simulink model "ControllerSimu"  (R2025b)
settings: Solver=VariableStepAuto  StartTime=0.0  StopTime=10.0  RelTol=1e-3
undefined symbols (not defined in the file or in its folder): a, b, delta_bp, Iz, TWFront, TWRear, U_bp, WheelRadius, Yaw_table
settings Model: Creator=ATuck  LastModifiedBy=ATuck

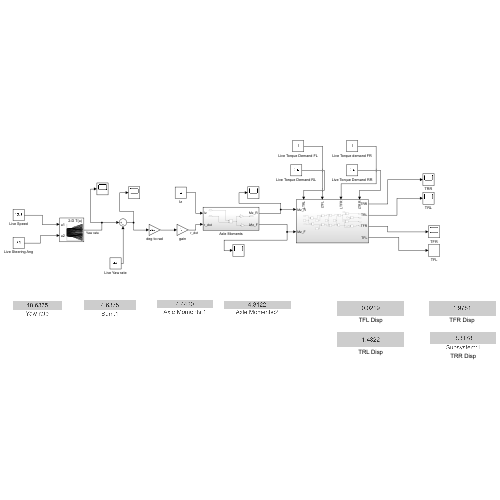
[thumbnail: Simulink's stored preview of the top-level diagram]
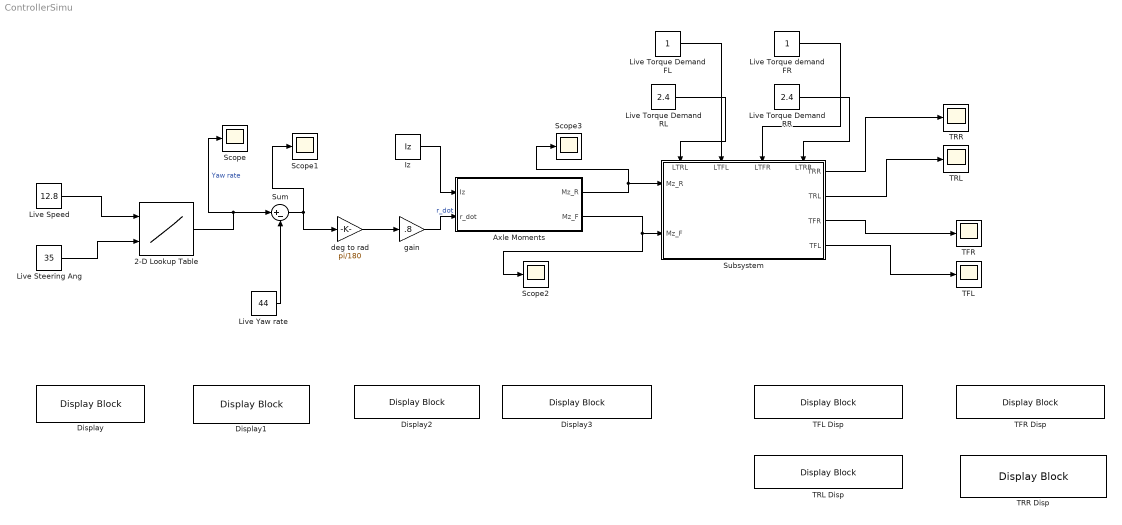
== system ControllerSimu ==
  2-D Lookup Table : Lookup_n-D  LookupTableObject=yaw_table  BreakpointsForDimension1=U_bp  BreakpointsForDimension2=delta_bp  Table=Yaw_table  InternalRulePriority=Speed  RndMeth=Simplest
      settings: InputPortMap=u0,u1
  Axle Moments : Subsystem
  Display{,1..3} (4 alike) : DisplayBlock  LabelPosition=Bottom  Transparency=1  GridColor=[0.502, 0.502, 0.502]
  Iz : Constant  Value=Iz
  Live Speed : Constant  Value=12.8
  Live Steering Ang : Constant  Value=35
  Live Torque Demand FL : Constant
  Live Torque Demand RL : Constant  Value=2.4
  Live Torque Demand RR : Constant  Value=2.4
  Live Torque demand FR : Constant
  Live Yaw rate : Constant  Value=44
  Scope{,1..3} (4 alike) : Scope
      Scope2 settings: DataLoggingVariableName=ScopeData2
      Scope3 settings: DataLoggingVariableName=ScopeData3
  Subsystem : Subsystem
      settings: PortSchema="{\"entries\":[{\"content\":{\"sides\":[{\"content\":{\"connectorIds\":[\"In1\",\"In2\"]},\"type\":\"ConnectorPlacement.EquallySpacedRectSide\",\"uuid\":\"e4f385be-e286-4044-9303-1c3b16f4ddb6\"},{\"content\":{\"connectorIds\":[\"Out1\",\"Out2\",\"Out3\",\"Out4\"],\"side\":\"RIGHT\"},\"type\":\"ConnectorPlacement.EquallySpacedRectSide\",\"uuid\":\"483c36ee-ea33-4761-a024-168230838bcf\"},{\"content\":{\"connectorIds\":[\"In3\",\"In4\",\"In5\",\"In6\"],\"side\":\"TOP\"},\"type\":\"ConnectorPlacement.EquallySpacedRectSide\",\"uuid\":\"c663e4d8-6ff0-495b-b829-be4485670536\"}]},\"type\":\"ConnectorPlacement.EquallySpacedConnector\",\"uuid\":\"2108b5a4-3d1e-4aea-a044-b4d481144d8a\"}],\"packageUris\":[\"http://schema.mathworks.com/mf0/Connector/R2020b\"],\"version\":\"1.0\"}"
  Sum : Sum  Inputs=|+-
  TFL : Scope
      settings: DataLoggingVariableName=ScopeData7
  TFL Disp : DisplayBlock  LabelPosition=Hide  Transparency=1  GridColor=[0.502, 0.502, 0.502]
  TFR : Scope
      settings: ActiveDisplayYMinimum=0.978093293694583  ActiveDisplayYMaximum=2.9780932936945828  DataLoggingVariableName=ScopeData6
  TFR Disp : DisplayBlock  LabelPosition=Hide  Transparency=1  GridColor=[0.502, 0.502, 0.502]
  TRL : Scope
      settings: DataLoggingVariableName=ScopeData5
  TRL Disp : DisplayBlock  LabelPosition=Hide  Transparency=1  GridColor=[0.502, 0.502, 0.502]
  TRR : Scope
      settings: DataLoggingVariableName=ScopeData4
  TRR Disp : DisplayBlock  LabelPosition=Bottom  Transparency=1  GridColor=[0.502, 0.502, 0.502]
  deg to rad : Gain  Gain=pi/180
  gain : Gain  Gain=.8
  wires:
  Live Speed/1 -> 2-D Lookup Table/1
  Live Steering Ang/1 -> 2-D Lookup Table/2
  Live Yaw rate/1 -> Sum/2
  Sum/1 -> deg to rad/1, Scope1/1
  Iz/1 -> Axle Moments/1(Iz)
  2-D Lookup Table/1 -> Sum/1, Scope/1  "Yaw rate"
  Axle Moments/2(Mz_F) -> Scope2/1, Subsystem/2(Mz_F)
  Axle Moments/1(Mz_R) -> Scope3/1, Subsystem/1(Mz_R)
  Live Torque Demand RL/1 -> Subsystem/3(LTRL)
  Live Torque Demand RR/1 -> Subsystem/6(LTRR)
  Live Torque Demand FL/1 -> Subsystem/4(LTFL)
  Live Torque demand FR/1 -> Subsystem/5(LTFR)
  Subsystem/1(TRR) -> TRR/1
  Subsystem/2(TRL) -> TRL/1
  Subsystem/3(TFR) -> TFR/1
  Subsystem/4(TFL) -> TFL/1
  deg to rad/1 -> gain/1
  gain/1 -> Axle Moments/2(r_dot)  "r_dot"

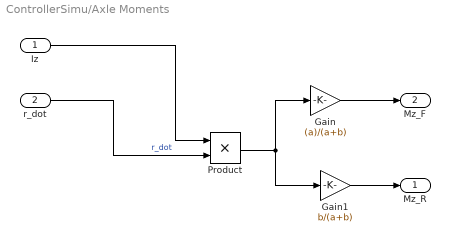
== system ControllerSimu/Axle Moments ==
  Iz : Inport
  r_dot : Inport  Port=2
  Gain : Gain  Gain=(a)/(a+b)
  Gain1 : Gain  Gain=b/(a+b)
  Product : Product
  Mz_R : Outport
  Mz_F : Outport  Port=2
  wires:
  r_dot/1 -> Product/2  "r_dot"
  Iz/1 -> Product/1
  Product/1 -> Gain1/1, Gain/1
  Gain1/1 -> Mz_R/1
  Gain/1 -> Mz_F/1

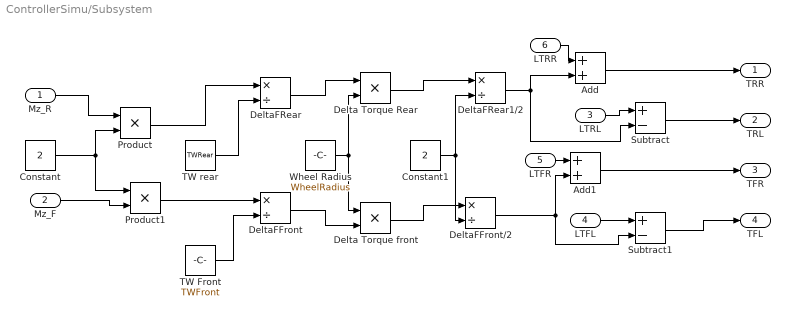
== system ControllerSimu/Subsystem ==
  Mz_R : Inport
  Mz_F : Inport  Port=2
  LTRL : Inport  Port=3
  LTFL : Inport  Port=4
  LTFR : Inport  Port=5
  LTRR : Inport  Port=6
  Add : Sum
  Add1 : Sum
  Constant : Constant  Value=2
  Constant1 : Constant  Value=2
  Delta Torque Rear : Product
  Delta Torque front : Product
  DeltaFFront : Product  Inputs=*/
  DeltaFFront/2 : Product  Inputs=*/
  DeltaFRear : Product  Inputs=*/
  DeltaFRear1/2 : Product  Inputs=*/
  Product : Product
  Product1 : Product
  Subtract : Sum  Inputs=+-
  Subtract1 : Sum  Inputs=+-
  TW Front : Constant  Value=TWFront
  TW rear : Constant  Value=TWRear
  Wheel Radius : Constant  Value=WheelRadius
  TRR : Outport
  TRL : Outport  Port=2
  TFR : Outport  Port=3
  TFL : Outport  Port=4
  wires:
  Mz_R/1 -> Product/1
  Constant/1 -> Product/2, Product1/1
  Mz_F/1 -> Product1/2
  Product/1 -> DeltaFRear/1
  Product1/1 -> DeltaFFront/1
  TW rear/1 -> DeltaFRear/2
  TW Front/1 -> DeltaFFront/2
  DeltaFFront/1 -> Delta Torque front/2
  DeltaFRear/1 -> Delta Torque Rear/1
  Wheel Radius/1 -> Delta Torque front/1, Delta Torque Rear/2
  Constant1/1 -> DeltaFFront/2/2, DeltaFRear1/2/2
  Delta Torque front/1 -> DeltaFFront/2/1
  Delta Torque Rear/1 -> DeltaFRear1/2/1
  LTRL/1 -> Subtract/1
  DeltaFRear1/2/1 -> Add/2, Subtract/2
  LTFL/1 -> Subtract1/1
  DeltaFFront/2/1 -> Subtract1/2, Add1/2
  LTRR/1 -> Add/1
  LTFR/1 -> Add1/1
  Add/1 -> TRR/1
  Subtract/1 -> TRL/1
  Subtract1/1 -> TFL/1
  Add1/1 -> TFR/1
